simulink model "IFSSIM_Chassis"  (R2025b)
settings: Solver=FixedStepDiscrete  StartTime=0  StopTime=inf  FixedStep=1/960  RelTol=1e-3
undefined symbols (not defined in the file): IFSSIM_PoseBus_zero
settings Model: Creator=raulmoran  LastModifiedBy=raulmoran

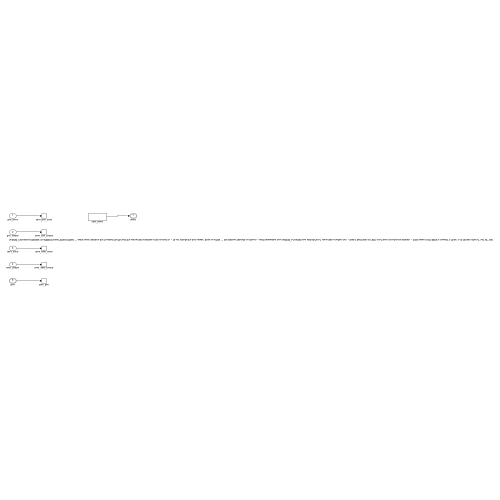
[thumbnail: Simulink's stored preview of the top-level diagram]
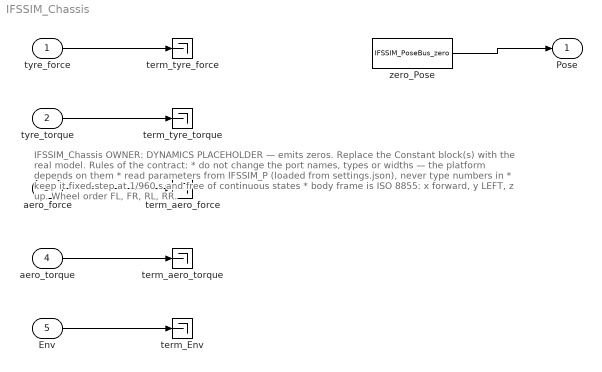
== system IFSSIM_Chassis ==
  note: IFSSIM_Chassis\n\nOWNER: DYNAMICS\n\nPLACEHOLDER — emits zeros. Replace the Constant block(s) with the real model.\n\nRules of the contract:\n * do not change the port names, types or widths — the platform depends on them\n * read parameters from IFSSIM_P (loaded from settings.json), never type numbers in\n * keep it fixed-step at 1/960 s and free of continuous states\n * body frame is ISO 8855: x forward, y LEFT, z up. Wheel order FL, FR, RL, RR.
  tyre_force : Inport  PortDimensions=3
  tyre_torque : Inport  Port=2  PortDimensions=3
  aero_force : Inport  Port=3  PortDimensions=3
  aero_torque : Inport  Port=4  PortDimensions=3
  Env : Inport  Port=5  OutDataTypeStr=Bus: IFSSIM_EnvBus  BusOutputAsStruct=on
  term_Env : Terminator
  term_aero_force : Terminator
  term_aero_torque : Terminator
  term_tyre_force : Terminator
  term_tyre_torque : Terminator
  zero_Pose : Constant  Value=IFSSIM_PoseBus_zero  OutDataTypeStr=Bus: IFSSIM_PoseBus
  Pose : Outport  OutDataTypeStr=Bus: IFSSIM_PoseBus
  wires:
  tyre_force/1 -> term_tyre_force/1
  tyre_torque/1 -> term_tyre_torque/1
  aero_force/1 -> term_aero_force/1
  aero_torque/1 -> term_aero_torque/1
  Env/1 -> term_Env/1
  zero_Pose/1 -> Pose/1
